simulink model "oke_qudus"  (R2023b)
settings: Solver=VariableStepAuto  StartTime=0.0  StopTime=10.0  RelTol=1e-3
values from neighbouring files (symbols this model uses):
  Bt = 0.0869    [dc_machine_control_1.m]
  Hc = 0.355    [dc_machine_control_1.m]
  J = 0.0607    [dc_machine_control_1.m]
  Kb = 1.26    [dc_machine_control_1.m]
  Kc = 2.33    [dc_machine_control_1.m]
  Kr = 31.05    [dc_machine_control_1.m]
  Ks = 28.73    [dc_machine_control_1.m]
  Kw = 0.065    [dc_machine_control_1.m]
  La = 0.072    [dc_machine_control_1.m]
  Ra = 4    [dc_machine_control_1.m]
  Tc = 0.0208    [dc_machine_control_1.m]
  Tr = 0.00138    [dc_machine_control_1.m]
  Ts = 0.0188    [dc_machine_control_1.m]
  Tw = 0.002    [dc_machine_control_1.m]
settings Model: Creator=USER  LastModifiedBy=USER

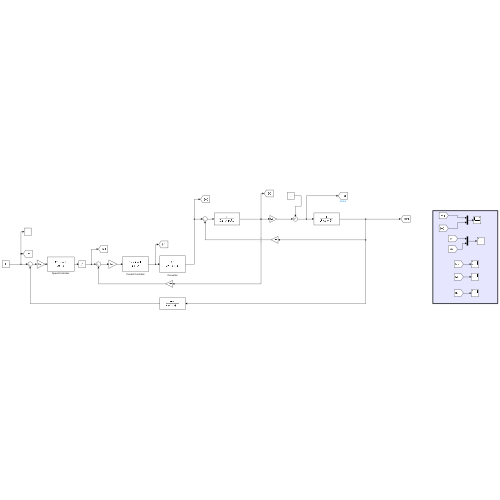
[thumbnail: Simulink's stored preview of the top-level diagram]
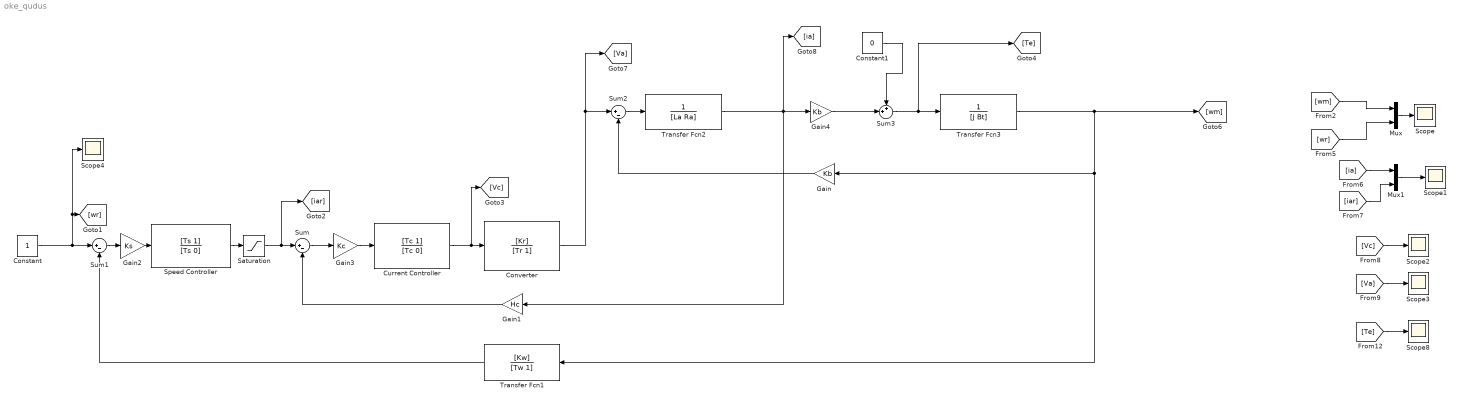
== system oke_qudus ==
  Constant : Constant
  Constant1 : Constant  Value=0
  Converter : TransferFcn  Numerator=[Kr]  Denominator=[Tr 1]
  Current Controller : TransferFcn  Numerator=[Tc 1]  Denominator=[Tc 0]
  Gain : Gain  Gain=Kb
  Gain1 : Gain  Gain=Hc
  Gain2 : Gain  Gain=Ks
  Gain3 : Gain  Gain=Kc
  Gain4 : Gain  Gain=Kb
  Mux : Mux  Inputs=2
  Mux1 : Mux  Inputs=2
  Saturation : Saturate  UpperLimit=10  LowerLimit=0
  Scope{,1..4,8} (6 alike) : Scope
  Speed Controller : TransferFcn  Numerator=[Ts 1]  Denominator=[Ts 0]
  Sum : Sum  Inputs=|+-
  Sum1 : Sum  Inputs=|+-
  Sum2 : Sum  Inputs=|+-
  Sum3 : Sum  Inputs=++|
  Transfer Fcn1 : TransferFcn  Numerator=[Kw]  Denominator=[Tw 1]
  Transfer Fcn2 : TransferFcn  Denominator=[La Ra]
  Transfer Fcn3 : TransferFcn  Denominator=[J Bt]
  wires:
  Sum/1 -> Gain3/1
  Transfer Fcn1/1 -> Sum1/2
  Constant/1 -> Scope4/1, [wr], Sum1/1
  Current Controller/1 -> Converter/1, [Vc]
  Gain3/1 -> Current Controller/1
  Saturation/1 -> Sum/1, [iar]
  Speed Controller/1 -> Saturation/1
  Sum1/1 -> Gain2/1
  Gain1/1 -> Sum/2
  Gain2/1 -> Speed Controller/1
  Gain4/1 -> Sum3/2
  Gain/1 -> Sum2/2
  Transfer Fcn2/1 -> Gain1/1, [ia], Gain4/1
  Converter/1 -> [Va], Sum2/1
  Sum3/1 -> [Te], Transfer Fcn3/1
  Constant1/1 -> Sum3/1
  Sum2/1 -> Transfer Fcn2/1
  Transfer Fcn3/1 -> Gain/1, Transfer Fcn1/1, [wm]
  [wr] -> Mux/2
  [Te] -> Scope8/1
  [iar] -> Mux1/2
  Mux1/1 -> Scope1/1
  [Vc] -> Scope2/1
  Mux/1 -> Scope/1
  [wm] -> Mux/1
  [ia] -> Mux1/1
  [Va] -> Scope3/1
